simulink model "Synapse"  (R2019a)
settings: Solver=VariableStepAuto  StartTime=0.0  StopTime=testtime  RelTol=1e-3
InitFcn:
  | Synapse_Test_Parameters
StopFcn:
  | Verify_Synapse
values from neighbouring files (symbols this model uses):
  alpha1 = 1.5e-6*100e3    (= 0.15)    [Synapse_Test_Parameters.m]
  alpha2 = 1e-2*100e3    (= 1000)    [Synapse_Test_Parameters.m]
  cf_factor = min(cfsat, 10^(cfslope*cf/1e3 + cfconst)) * 2.0    [Synapse_Test_Parameters.m]
  Fs = 48e3    (= 48000)    [Synapse_Test_Parameters.m]
  multFac = max(2.95*max(1.0,1.5-spont/100), 4.3-0.2*cf/1e3)    [Synapse_Test_Parameters.m]
  nSites = 4    [Synapse_Test_Parameters.m]
  spont = 100    [Synapse_Test_Parameters.m]
  tabs = 0.6e-3    (= 0.0006)    [Synapse_Test_Parameters.m]
  tdres = 1/Fs    (= 2.08333333333e-05)    [Synapse_Test_Parameters.m]
  trel = 0.6e-3    (= 0.0006)    [Synapse_Test_Parameters.m]
undefined symbols (not defined in the file or in its folder): dfilt
libraries: dspsrcs4 x3, dsparch4 x2
(part 1 of 2)
settings Model: NumberOfSteps=50  Creator=mblun  LastModifiedBy=mblun

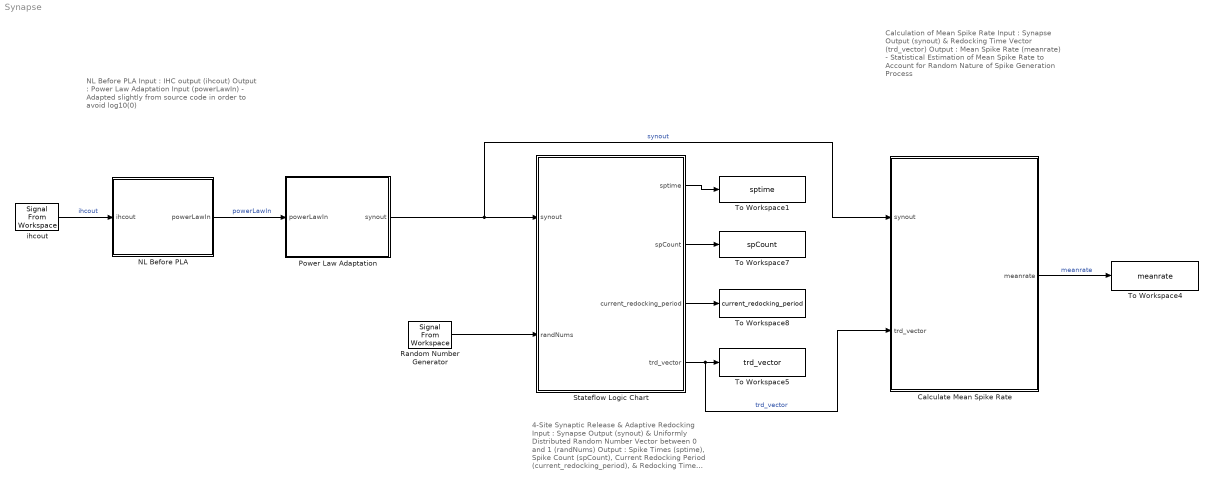
== system Synapse ==
  note: NL Before PLA
      |
      | Input : IHC output (ihcout)
      |
      | Output : Power Law Adaptation Input (powerLawIn)
      |
      | - Adapted slightly from source code in order to avoid log10(0)
  note: 4-Site Synaptic Release & Adaptive Redocking
      |
      | Input : Synapse Output (synout) & Uniformly Distributed Random Number Vector between 0 and 1 (randNums)
      |
      | Output : Spike Times (sptime), Spike Count (spCount), Current Redocking Period (current_redocking_period), & Redocking Time Vector (trd_vector)
      |
      | - Implemented using Stateflow Chart and embedded MATLAB functions
      |
      | - Shows states of synaptic sites during simulation
  note: Calculation of Mean Spike Rate
      |
      | Input : Synapse Output (synout) & Redocking Time Vector (trd_vector)
      |
      | Output : Mean Spike Rate (meanrate)
      |
      | - Statistical Estimation of Mean Spike Rate to Account for Random Nature of Spike Generation Process
  Calculate Mean Spike Rate : Subsystem
  NL Before PLA : Subsystem
  Power Law Adaptation : Subsystem
  Random Number Generator : dspsrcs4/Signal From Workspace  X=randNums  Ts=1/Fs  nsamps=1  OutputAfterFinalValue=Setting to zero  ignoreOrWarnInputAndFrameLengths=off  OutputFrames=off
  Stateflow Logic Chart : Stateflow chart  BlockKeywords=__PRM__SERIALIZED__DATA__:Stateflow Chart,Stateflow Diagram  TreatAsAtomicUnit=on
  To Workspace1 : ToWorkspace  VariableName=sptime  SampleTime=-1
      settings: Save2DSignal=2-D array (concatenate along first dimension)
  To Workspace4 : ToWorkspace  VariableName=meanrate  SampleTime=-1
      settings: Save2DSignal=2-D array (concatenate along first dimension)
  To Workspace5 : ToWorkspace  VariableName=trd_vector  SampleTime=-1
      settings: Save2DSignal=2-D array (concatenate along first dimension)
  To Workspace7 : ToWorkspace  VariableName=spCount  SampleTime=-1
      settings: Save2DSignal=2-D array (concatenate along first dimension)
  To Workspace8 : ToWorkspace  VariableName=current_redocking_period  SampleTime=-1
      settings: Save2DSignal=2-D array (concatenate along first dimension)
  ihcout : dspsrcs4/Signal From Workspace  X=RxSignal  Ts=tdres  nsamps=1  OutputAfterFinalValue=Setting to zero  ignoreOrWarnInputAndFrameLengths=off  OutputFrames=off
  wires:
  Power Law Adaptation/1(synout) -> Stateflow Logic Chart/1(synout), Calculate Mean Spike Rate/1(synout)  "synout"
  ihcout/1 -> NL Before PLA/1(ihcout)  "ihcout"
  NL Before PLA/1(powerLawIn) -> Power Law Adaptation/1(powerLawIn)  "powerLawIn"
  Calculate Mean Spike Rate/1(meanrate) -> To Workspace4/1  "meanrate"
  Stateflow Logic Chart/3(current_redocking_period) -> To Workspace8/1
  Stateflow Logic Chart/1(sptime) -> To Workspace1/1
  Stateflow Logic Chart/4(trd_vector) -> Calculate Mean Spike Rate/2(trd_vector), To Workspace5/1  "trd_vector"
  Stateflow Logic Chart/2(spCount) -> To Workspace7/1
  Random Number Generator/1 -> Stateflow Logic Chart/2(randNums)

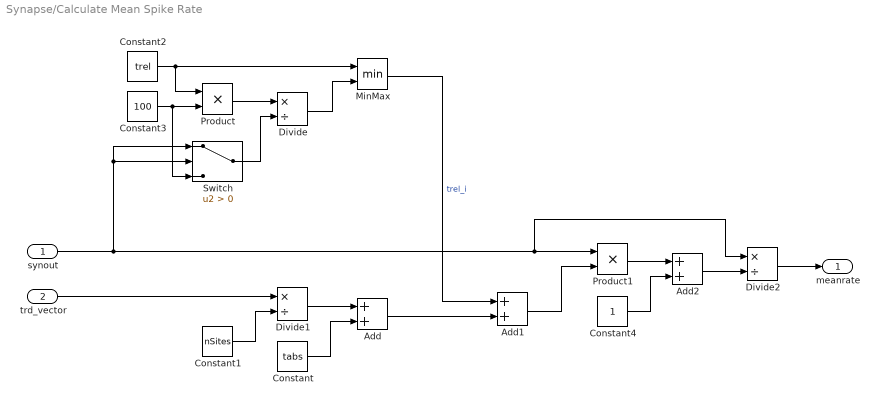
== system Synapse/Calculate Mean Spike Rate ==
  synout : Inport
  trd_vector : Inport  Port=2
  Add : Sum
  Add1 : Sum
  Add2 : Sum
  Constant : Constant  Value=tabs  SampleTime=-1
  Constant1 : Constant  Value=nSites  SampleTime=-1
  Constant2 : Constant  Value=trel  SampleTime=-1
  Constant3 : Constant  Value=100  SampleTime=-1
  Constant4 : Constant  SampleTime=-1
  Divide : Product  Inputs=*/  SaturateOnIntegerOverflow=on  RndMeth=Zero
  Divide1 : Product  Inputs=*/  SaturateOnIntegerOverflow=on  RndMeth=Zero
  Divide2 : Product  Inputs=*/  SaturateOnIntegerOverflow=on  RndMeth=Zero
  MinMax : MinMax  Inputs=2
  Product : Product
  Product1 : Product
  Switch : Switch  Criteria=u2 > Threshold
  meanrate : Outport
  wires:
  synout/1 -> Switch/1, Switch/2, Divide2/1, Product1/1
  trd_vector/1 -> Divide1/1
  Constant2/1 -> MinMax/1, Product/1
  Constant3/1 -> Switch/3, Product/2
  Product/1 -> Divide/1
  Divide/1 -> MinMax/2
  MinMax/1 -> Add1/1  "trel_i"
  Constant1/1 -> Divide1/2
  Divide1/1 -> Add/1
  Constant/1 -> Add/2
  Add/1 -> Add1/2
  Constant4/1 -> Add2/2
  Add1/1 -> Product1/2
  Product1/1 -> Add2/1
  Add2/1 -> Divide2/2
  Divide2/1 -> meanrate/1
  Switch/1 -> Divide/2

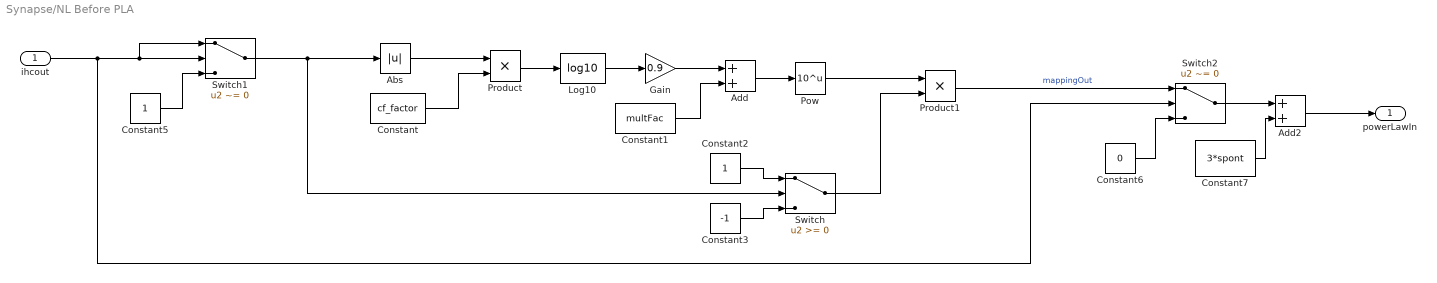
== system Synapse/NL Before PLA ==
  ihcout : Inport
  Abs : Abs
  Add : Sum
  Add2 : Sum
  Constant : Constant  Value=cf_factor  SampleTime=-1
  Constant1 : Constant  Value=multFac  SampleTime=-1
  Constant2 : Constant  SampleTime=-1
  Constant3 : Constant  Value=-1  SampleTime=-1
  Constant5 : Constant  SampleTime=-1
  Constant6 : Constant  Value=0  SampleTime=-1
  Constant7 : Constant  Value=3*spont  SampleTime=-1
  Gain : Gain  Gain=0.9
  Log10 : Math  Operator=log10  RndMeth=Zero  SaturateOnIntegerOverflow=on
  Pow : Math  Operator=10^u  RndMeth=Zero  SaturateOnIntegerOverflow=on
  Product : Product
  Product1 : Product
  Switch : Switch
  Switch1 : Switch  Criteria=u2 ~= 0
  Switch2 : Switch  Criteria=u2 ~= 0
  powerLawIn : Outport
  wires:
  Constant/1 -> Product/2
  Abs/1 -> Product/1
  Product/1 -> Log10/1
  Log10/1 -> Gain/1
  Gain/1 -> Add/1
  Constant1/1 -> Add/2
  Add/1 -> Pow/1
  Constant3/1 -> Switch/3
  Constant2/1 -> Switch/1
  Pow/1 -> Product1/1
  Switch/1 -> Product1/2
  Product1/1 -> Switch2/1  "mappingOut"
  Switch1/1 -> Abs/1, Switch/2
  ihcout/1 -> Switch2/2, Switch1/1, Switch1/2
  Constant5/1 -> Switch1/3
  Constant6/1 -> Switch2/3
  Switch2/1 -> Add2/1
  Constant7/1 -> Add2/2
  Add2/1 -> powerLawIn/1

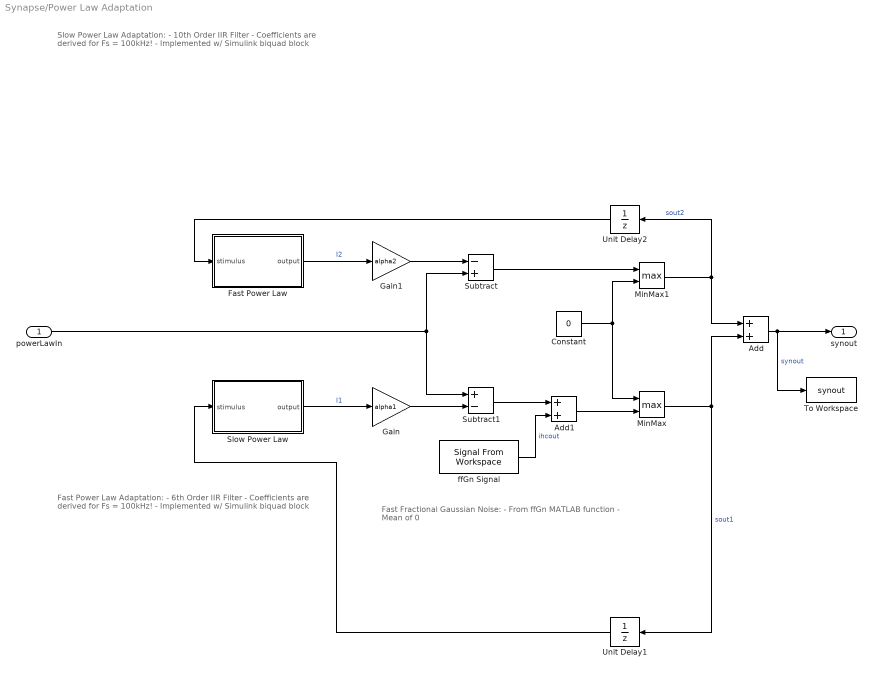
== system Synapse/Power Law Adaptation ==
  note: Fast Power Law Adaptation:
      |
      | - 6th Order IIR Filter
      |
      | - Coefficients are derived for Fs = 100kHz!
      |
      | - Implemented w/ Simulink biquad block
  note: Slow Power Law Adaptation:
      |
      | - 10th Order IIR Filter
      |
      | - Coefficients are derived for Fs = 100kHz!
      |
      | - Implemented w/ Simulink biquad block
  note: Fast Fractional Gaussian Noise:
      |
      | - From ffGn MATLAB function
      |
      | - Mean of 0
  powerLawIn : Inport
  Add : Sum
  Add1 : Sum
  Constant : Constant  Value=0  SampleTime=-1
  Fast Power Law : Subsystem
  Gain : Gain  Gain=alpha1
  Gain1 : Gain  Gain=alpha2
  MinMax : MinMax  Function=max  Inputs=2
  MinMax1 : MinMax  Function=max  Inputs=2
  Slow Power Law : Subsystem
  Subtract : Sum  Inputs=-+
  Subtract1 : Sum  Inputs=+-
  To Workspace : ToWorkspace  VariableName=synout  SampleTime=-1
      settings: Save2DSignal=2-D array (concatenate along first dimension)
  Unit Delay1 : UnitDelay  SampleTime=-1  HasFrameUpgradeWarning=on
  Unit Delay2 : UnitDelay  SampleTime=-1  HasFrameUpgradeWarning=on
  ffGn Signal : dspsrcs4/Signal From Workspace  X=noise  Ts=1/Fs  nsamps=1  OutputAfterFinalValue=Setting to zero  ignoreOrWarnInputAndFrameLengths=off  OutputFrames=off
  synout : Outport
  wires:
  Gain/1 -> Subtract1/2
  Subtract/1 -> MinMax1/1
  MinMax1/1 -> Unit Delay2/1, Add/1  "sout2"
  Add/1 -> synout/1, To Workspace/1  "synout"
  powerLawIn/1 -> Subtract/2, Subtract1/1
  Fast Power Law/1(output) -> Gain1/1  "I2"
  Unit Delay2/1 -> Fast Power Law/1(stimulus)
  Slow Power Law/1(output) -> Gain/1  "I1"
  Subtract1/1 -> Add1/1
  Constant/1 -> MinMax/1, MinMax1/2
  MinMax/1 -> Unit Delay1/1, Add/2  "sout1"
  Unit Delay1/1 -> Slow Power Law/1(stimulus)
  Gain1/1 -> Subtract/1
  Add1/1 -> MinMax/2
  ffGn Signal/1 -> Add1/2  "ihcout"

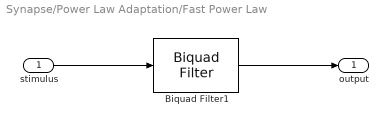
== system Synapse/Power Law Adaptation/Fast Power Law ==
  stimulus : Inport
  Biquad Filter1 : dsparch4/Biquad Filter  FilterSource=Dialog parameters  CoeffSource=Specify via dialog  FilterObject=dfilt.df2tsos([1 0.3 0.4],[1 0.1 0.2])  IIRFiltStruct=Direct form I  BiQuadCoeffs=fast_coeffs  ScaleValues=1  IC=0  ICnum=0  ICden=0  a0Flag=Warning  optimizeScaleValues=on  ScaleValueMode=Specify via input port (g)  roundingMode=Floor  overflowMode=on  scaleValueFracLength=14  denProdOutputFracLength=30  denAccumFracLength=30  secondMemoryFracLength=15
      settings: SourceProductName=DSP System Toolbox
  output : Outport
  wires:
  stimulus/1 -> Biquad Filter1/1
  Biquad Filter1/1 -> output/1

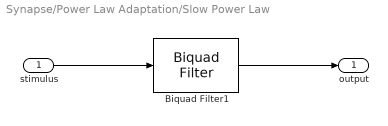
== system Synapse/Power Law Adaptation/Slow Power Law ==
  stimulus : Inport
  Biquad Filter1 : dsparch4/Biquad Filter  FilterSource=Dialog parameters  CoeffSource=Specify via dialog  FilterObject=dfilt.df2tsos([1 0.3 0.4],[1 0.1 0.2])  IIRFiltStruct=Direct form I  BiQuadCoeffs=slow_coeffs  ScaleValues=1  IC=0  ICnum=0  ICden=0  a0Flag=Warning  optimizeScaleValues=on  ScaleValueMode=Specify via input port (g)  roundingMode=Floor  overflowMode=on  scaleValueFracLength=14  denProdOutputFracLength=30  denAccumFracLength=30  secondMemoryFracLength=15
      settings: SourceProductName=DSP System Toolbox
  output : Outport
  wires:
  stimulus/1 -> Biquad Filter1/1
  Biquad Filter1/1 -> output/1
